simulink model "kp"  (Simulink 8.5)
settings: Solver=ode23tb  StartTime=0.0  StopTime=10  MaxStep=10e-6  RelTol=1e-3
InitFcn:
  | fs=1000;
libraries: powerlib x8, simulink x3, re_lib x1
settings Model: Creator=KASHIF  LastModifiedBy=Administrador
settings DebuggingCC: SolverPrmCheckMsg=warning  FcnCallInpInsideContextMsg=UseLocalSettings

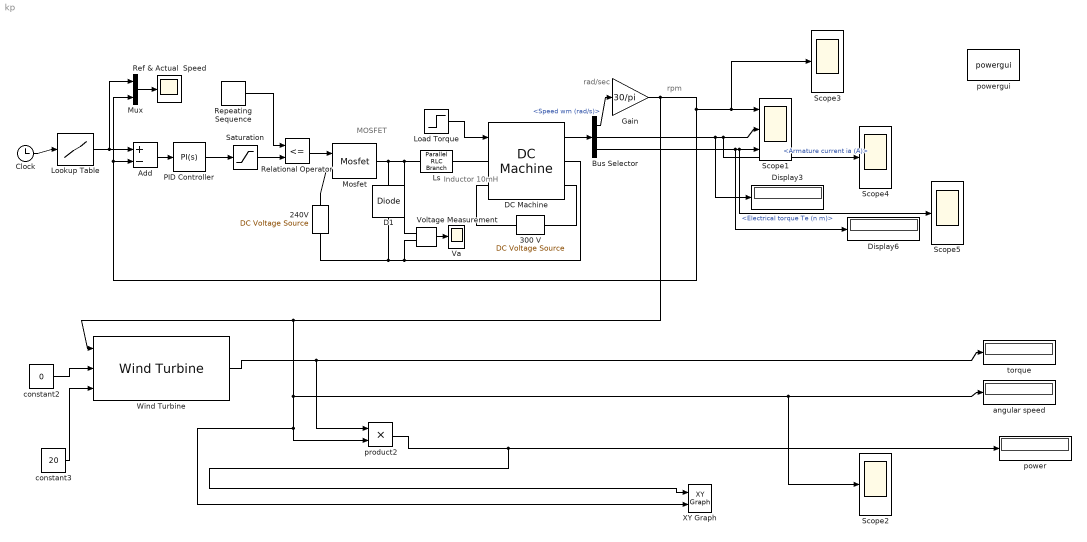
== system kp ==
  note: Inductor 10mH
  note: rad/sec
  note: rpm
  note: MOSFET
  "240V " : powerlib/Electrical Sources/DC Voltage Source  Description=source block  Amplitude=240  Measurements=None
      settings: AttributesFormatString=\n
  300 V : powerlib/Electrical Sources/DC Voltage Source  Description=source block  Amplitude=300  Measurements=None
      settings: AttributesFormatString=\n
  Add : Sum  Inputs=+-
  Bus Selector : BusSelector  OutputSignals=Speed wm (rad/s),Armature current ia (A),Electrical torque Te (n m)
  Clock : Clock
  D1 : powerlib/Power Electronics/Diode  Ron=0.05  Lon=0  Vf=0.7  IC=0  UseSnubber=off  Rs=Inf  Cs=0.1e-6  Measurements=off
  DC Machine : powerlib/Machines/DC Machine  PresetModel=01: 5HP 240V 1750RPM Field:300V  MechanicalLoad=Torque TL  FieldType=Wound  ShowDetailedParameters=on  MeasurementBus=off  RLa=[2.581 0.028]  RLf=[281.3 156]  Laf=0.9483  MachineConstant=Torque constant (N.m/A)  Ke=1.8  Kt=1.8  J=0.02215  Bm=0.002953  Tf=0.5161  w0=1  Ifinit=1  TsPowergui=0  TsBlock=-1
      settings: AttributesFormatString=\n
  Display3 : Display
  Display6 : Display
  Gain : Gain  Gain=30/pi
  Load Torque : Step  Time=0.75  After=10  SampleTime=0
  Lookup Table : Lookup  InputValues=[0 0.5 1.0 1.1 1.5 1.6 2 2.1 2.5]  Table=[0 1000 1000 850 850 1500 1500 500 500]
  Ls : powerlib/Elements/Parallel RLC Branch  LConnTagsString=a  RConnTagsString=__new0  BranchType=L  Resistance=1.0  Inductance=10e-03  SetiL0=off  InitialCurrent=0  Capacitance=1.0  Setx0=off  InitialVoltage=0  Measurements=None
  Mosfet : powerlib/Power Electronics/Mosfet  Ron=0.1  Lon=0  Rd=0.01  Vfd=0  IC=0  Rs=1e5  Cs=inf  Measurements=off
  Mux : Mux  Inputs=2
  PID Controller : simulink/Continuous/PID Controller  Controller=PI  TimeDomain=Continuous-time  SampleTime=-1  IntegratorMethod=Forward Euler  FilterMethod=Forward Euler  Form=Parallel  UseFilter=on  ControllerParametersSource=internal  P=0.001  I=0.02  D=0.0001  N=100  InitialConditionSource=internal  InitialConditionForIntegrator=0  InitialConditionForFilter=0  ExternalReset=none  LimitOutput=off  UpperSaturationLimit=inf  LowerSaturationLimit=-inf  LinearizeAsGain=off  AntiWindupMode=none  Kb=1  TrackingMode=off  Kt=1  PParamMin=[]  PParamMax=[]  IParamMin=[]  IParamMax=[]  DParamMin=[]  DParamMax=[]  NParamMin=[]  NParamMax=[]  KbParamMin=[]  KbParamMax=[]  KtParamMin=[]  KtParamMax=[]  POutMin=[]  POutMax=[]  IOutMin=[]  IOutMax=[]  DOutMin=[]  DOutMax=[]  NOutMin=[]  NOutMax=[]  KbOutMin=[]  KbOutMax=[]  KtOutMin=[]  KtOutMax=[]  IntegratorOutMin=[]  IntegratorOutMax=[]  FilterOutMin=[]  FilterOutMax=[]  SumOutMin=[]  SumOutMax=[]  SumI1OutMin=[]  SumI1OutMax=[]  SumI2OutMin=[]  SumI2OutMax=[]  SumI3OutMin=[]  SumI3OutMax=[]  SumDOutMin=[]  SumDOutMax=[]  SaturationOutMin=[]  SaturationOutMax=[]  IntegratorContinuousStateAttributes=''  IntegratorStateMustResolveToSignalObject=off  IntegratorRTWStateStorageClass=Auto  FilterContinuousStateAttributes=''  FilterStateMustResolveToSignalObject=off  FilterRTWStateStorageClass=Auto  DifferentiatorICPrevScaledInput=0  DifferentiatorOutMin=[]  DifferentiatorOutMax=[]
  Ref & Actual  Speed : Scope
      settings: YMin=0  YMax=1600  SaveName=ScopeData2  MaxDataPoints=5000000
  Relational Operator : RelationalOperator  Operator=<=  OutDataTypeStr=boolean
  Repeating Sequence : simulink/Sources/Repeating Sequence  rep_seq_t=[0 1/2000]  rep_seq_y=[0 1]
  Saturation : Saturate  UpperLimit=1  LowerLimit=0
  Scope1 : Scope  NumInputPorts=3
      settings: TimeRange=1  YMin=6.375~0.1~0.1  YMax=6.775~0.5~0.5  MaxDataPoints=5000000
  Scope{2..5} (4 alike) : Scope
      Scope2 settings: TimeRange=1  YMin=6.375  YMax=6.775  SaveName=ScopeData3  MaxDataPoints=5000000
      Scope3 settings: TimeRange=1  YMin=6.375  YMax=6.775  SaveName=ScopeData4  MaxDataPoints=5000000
      Scope4 settings: TimeRange=1  YMin=6.375  YMax=6.775  SaveName=ScopeData5  MaxDataPoints=5000000
      Scope5 settings: TimeRange=0.35  YMin=-1  YMax=7  SaveName=ScopeData6  MaxDataPoints=5000000
  Va : Scope
      settings: YMin=50  YMax=500  MaxDataPoints=5000000
  Voltage Measurement : powerlib/Measurements/Voltage Measurement  PhasorSimulation=off  OutputType=Complex  PSBequivalent=0
  Wind Turbine : re_lib/Wind Generation/Wind Turbine  Pnom=1.5e6  Pelec_base=1.5e6/0.9  wind_base=12  P_wind_base=0.73  speed_nom=1.2  pitch_angle=0  c1_c6="[0.51763          116          0.4            5           21     0.006795]"  cp_nom=0.48  lambda_nom=8.1
  XY Graph : simulink/Sinks/XY Graph  xmin=0  xmax=100  ymin=0  ymax=200  st=20
  angular speed : Display
  constant2 : Constant  Value=0
  constant3 : Constant  Value=20
  power : Display
  powergui : powerlib/powergui  Priority=1  SimulationMode=Continuous  SolverType=Tustin/Backward Euler (TBE)  SampleTime=50e-6  frequency=60  SPID=off  DisableSnubberDevices=off  DisableRonSwitches=off  DisableVfSwitches=off  SwTol=0  DisplayEquations=off  Interpol=off  methode=off  Ts=100  FunctionMessages=off  echomessages=off  HookPort=off  EnableUseOfTLC=off  x0status=blocks  frequencyindice=0  Pbase=100e6  ErrMax=1e-4  Iterations=50  UnitsV=kV  UnitsW=MW  buscounter=0  RestoreLinks=warning  ResistiveCurrentMeasurement=off  Frange=[0:2:500]  Ylog=off  Xlog=on  ShowGrid=off  save=off  variable=ZData  structure=0  ZoomFFT=off  StartTime=0.0  cycles=1  DisplayStyle=1  fundamental=60  FreqAxis=off  MaxFrequency=1000  frequencyindicesteady=1  RmsSteady=1  display=off
  product2 : Product  RndMeth=Zero
  torque : Display
  wires:
  Repeating Sequence/1 -> Relational Operator/1
  Relational Operator/1 -> Mosfet/1
  Load Torque/1 -> DC Machine/1
  DC Machine/1 -> Bus Selector/1
  Bus Selector/1 -> Gain/1  "<Speed wm (rad/s)>"
  Bus Selector/2 -> Display3/1, Scope1/2, Scope4/1  "<Armature current ia (A)>"
  Bus Selector/3 -> Display6/1, Scope1/3, Scope5/1  "<Electrical torque Te (n m)>"
  Gain/1 -> Wind Turbine/1, product2/2, XY Graph/2, Scope2/1, angular speed/1, Add/2, Mux/2, Scope1/1, Scope3/1
  Lookup Table/1 -> Add/1, Mux/1
  Add/1 -> PID Controller/1
  PID Controller/1 -> Saturation/1
  Saturation/1 -> Relational Operator/2
  Clock/1 -> Lookup Table/1
  Mux/1 -> Ref & Actual  Speed/1
  Voltage Measurement/1 -> Va/1
  Wind Turbine/1 -> torque/1, product2/1
  constant2/1 -> Wind Turbine/2
  constant3/1 -> Wind Turbine/3
  product2/1 -> XY Graph/1, power/1
  connections:
  Ls/LConn1 -- Voltage Measurement/LConn1 -- D1/RConn1 -- Mosfet/RConn1
  Ls/RConn1 -- DC Machine/LConn1
  300 V/RConn1 -- DC Machine/LConn2
  300 V/LConn1 -- DC Machine/RConn2
  "240V "/RConn1 -- Mosfet/LConn1
  DC Machine/RConn1 -- D1/LConn1 -- "240V "/LConn1 -- Voltage Measurement/LConn2
